simulink model "model_5"  (R2021a)
settings: Solver=VariableStepAuto  StartTime=0.0  StopTime=60.0  RelTol=1e-3
libraries: simulink x1
settings Model: Creator=mansi  LastModifiedBy=mansi

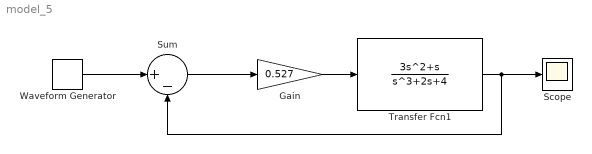
== system model_5 ==
  Gain : Gain  Gain=0.527
  Scope : Scope
  Sum : Sum  Inputs=|+-
  Transfer Fcn1 : TransferFcn  Numerator=[3,1,0]  Denominator=[1,0,2,4]
  Waveform Generator : simulink/Sources/Waveform Generator  OutMin=[]  OutMax=[]  OutDataTypeStr=double  SelectedSignal=1  Signals=step(0,0,1)  BlockNames=MultiportSwitch_77ad4a2251064ef  SampleTime=0.1
  wires:
  Waveform Generator/1 -> Sum/1
  Transfer Fcn1/1 -> Scope/1, Sum/2
  Sum/1 -> Gain/1
  Gain/1 -> Transfer Fcn1/1
